simulink model "Test_apparatus"  (R2017a)
settings: Solver=VariableStepAuto  StartTime=0.0  StopTime=10  FixedStep=0.00001  RelTol=1e-3
values from neighbouring files (symbols this model uses):
  b = 0    [Oct12workspace.mat]    (also in Test_apparatus_simulation.m; custom_sim.m = 2.134608e-06)
  J = 2.134608e-05    [Oct12workspace.mat]    (also in Test_apparatus_simulation.m; custom_sim.m)
  Kd = 1000    [Oct12workspace.mat]    (also in Test_apparatus_simulation.m = dd; bilat_teleop_time_delay_params.m = 0; custom_sim.m = 35; ode45_sim.m = 0)
  Ke = 0.142826110455    [Oct12workspace.mat]    (also in Test_apparatus_simulation.m; bilat_teleop_multiDOF_params.m = [0 0; 0 0]; sampled_data_bilat_teleop_tavakoli_params.m = 0; sampled_data_bilat_teleop_time_delay_params.m = 0)
  Kp = 10000    [Oct12workspace.mat]    (also in Test_apparatus_simulation.m = pp; bilat_teleop_time_delay_params.m = 0; custom_sim.m = 100; ode45_sim.m = 100)
  KpC = 375    [Oct12workspace.mat]    (also in Test_apparatus_simulation.m; custom_sim.m = 1)
  Kt = 0.0194    [Oct12workspace.mat]    (also in Test_apparatus_simulation.m)
  L = 8.5e-05    [Oct12workspace.mat]    (also in Test_apparatus_simulation.m; custom_sim.m)
  R = 0.314    [Oct12workspace.mat]    (also in Test_apparatus_simulation.m; custom_sim.m)
  Tcontrol = 0.001    [Oct12workspace.mat]    (also in Test_apparatus_simulation.m)
  VScale = 57.2957795131    [Oct12workspace.mat]    (also in Test_apparatus_simulation.m)
  XScale = 57.2957795131    [Oct12workspace.mat]    (also in Test_apparatus_simulation.m)
libraries: simulink x3
settings Model: Creator=sansh  LastModifiedBy=salou

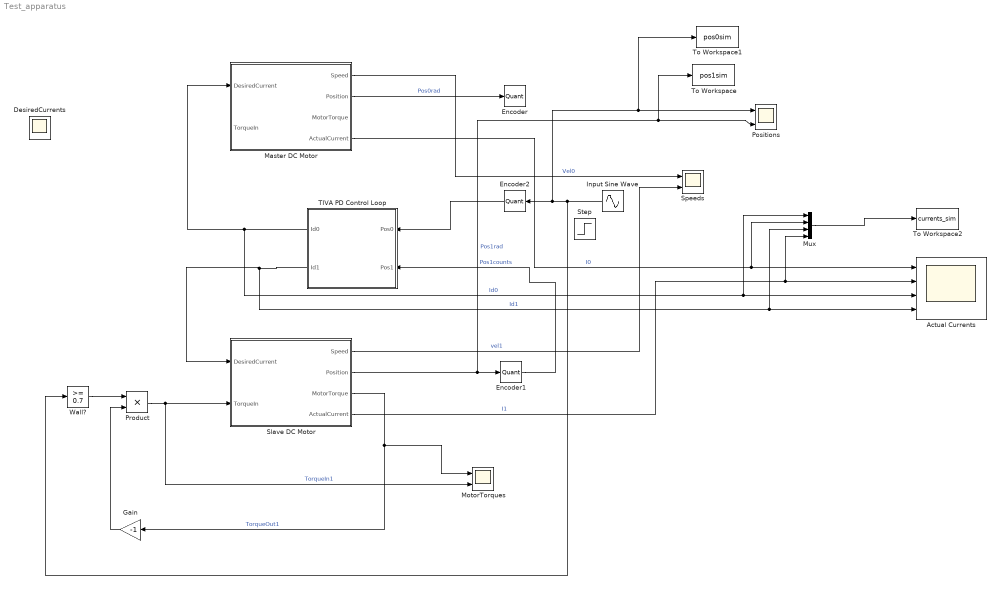
== system Test_apparatus ==
  Actual Currents : Scope  NumInputPorts=4
  DesiredCurrents : Scope
  Encoder : Quantizer  QuantizationInterval=(2*pi)/8192
  Encoder1 : Quantizer  QuantizationInterval=(2*pi)/8192
  Encoder2 : Quantizer  QuantizationInterval=(2*pi)/8192
  Gain : Gain  Gain=-1
  Input Sine Wave : Sin  SampleTime=0
  Master DC Motor : Subsystem
  MotorTorques : Scope  NumInputPorts=2
  Mux : Mux
  Positions : Scope  NumInputPorts=2
  Product : Product
  Slave DC Motor : Subsystem
  Speeds : Scope  NumInputPorts=2
  Step : Step  SampleTime=0
  TIVA PD Control Loop : Subsystem
  To Workspace : ToWorkspace  VariableName=pos1sim  SaveFormat=Timeseries  SampleTime=-1
  To Workspace1 : ToWorkspace  VariableName=pos0sim  SaveFormat=Timeseries  SampleTime=-1
  To Workspace2 : ToWorkspace  VariableName=currents_sim  SaveFormat=Timeseries  SampleTime=-1
  Wall? : simulink/Logic and Bit Operations/Compare To Constant  relop=>=  const=0.7  OutDataTypeStr=uint8
  wires:
  Master DC Motor/2(Position) -> Encoder/1  "Pos0rad"
  Slave DC Motor/2(Position) -> To Workspace/1, Positions/2, Encoder1/1  "Pos1rad"
  Encoder1/1 -> TIVA PD Control Loop/2(Pos1)  "Pos1counts"
  TIVA PD Control Loop/1(Id0) -> Mux/1, Actual Currents/3, Master DC Motor/1(DesiredCurrent)  "Id0"
  TIVA PD Control Loop/2(Id1) -> Slave DC Motor/1(DesiredCurrent), Mux/3, Actual Currents/4  "Id1"
  Input Sine Wave/1 -> Wall?/1, To Workspace1/1, Positions/1, Encoder2/1
  Encoder2/1 -> TIVA PD Control Loop/1(Pos0)
  Slave DC Motor/1(Speed) -> Speeds/2  "vel1"
  Master DC Motor/4(ActualCurrent) -> Mux/2, Actual Currents/1  "I0"
  Slave DC Motor/4(ActualCurrent) -> Mux/4, Actual Currents/2  "I1"
  Master DC Motor/1(Speed) -> Speeds/1  "Vel0"
  Mux/1 -> To Workspace2/1
  Wall?/1 -> Product/1
  Slave DC Motor/3(MotorTorque) -> MotorTorques/1, Gain/1  "TorqueOut1"
  Product/1 -> Slave DC Motor/2(TorqueIn), MotorTorques/2  "TorqueIn1"
  Gain/1 -> Product/2

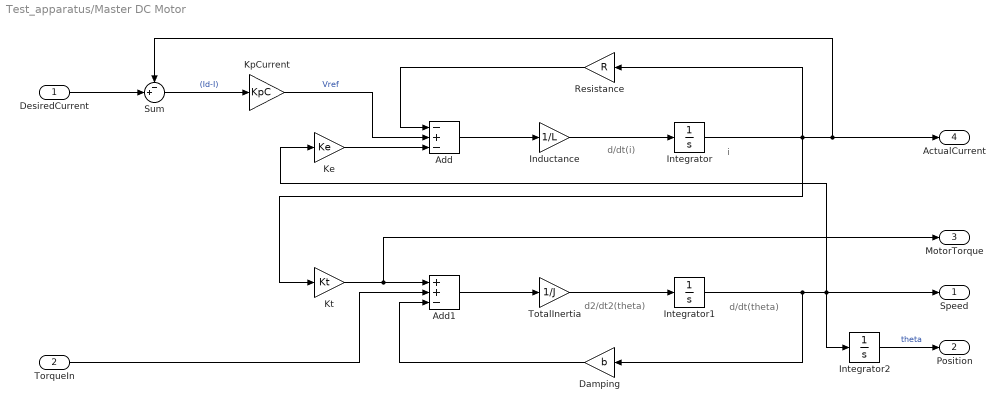
== system Test_apparatus/Master DC Motor ==
  note: i
  note: d/dt(i)
  note: d/dt(theta)
  note: d2/dt2(theta)
  DesiredCurrent : Inport
  TorqueIn : Inport  Port=2
  Add : Sum  Inputs=-+-
  Add1 : Sum  Inputs=++-
  Damping : Gain  Gain=b
  Inductance : Gain  Gain=1/L
  Integrator : Integrator
  Integrator1 : Integrator
  Integrator2 : Integrator
  Ke : Gain  Gain=Ke
  KpCurrent : Gain  Gain=KpC
  Kt : Gain  Gain=Kt
  Resistance : Gain  Gain=R
  Sum : Sum  Inputs=-+|
  TotalInertia : Gain  Gain=1/J
  Speed : Outport
  Position : Outport  Port=2
  MotorTorque : Outport  Port=3
  ActualCurrent : Outport  Port=4
  wires:
  Inductance/1 -> Integrator/1
  Integrator1/1 -> Damping/1, Integrator2/1, Speed/1, Ke/1
  TotalInertia/1 -> Integrator1/1
  Integrator/1 -> ActualCurrent/1, Sum/1, Resistance/1, Kt/1
  Kt/1 -> MotorTorque/1, Add1/1
  KpCurrent/1 -> Add/2  "Vref"
  Resistance/1 -> Add/1
  Damping/1 -> Add1/3
  Ke/1 -> Add/3
  Add/1 -> Inductance/1
  Add1/1 -> TotalInertia/1
  Integrator2/1 -> Position/1  "theta"
  DesiredCurrent/1 -> Sum/2
  Sum/1 -> KpCurrent/1  "(Id-I)"
  TorqueIn/1 -> Add1/2

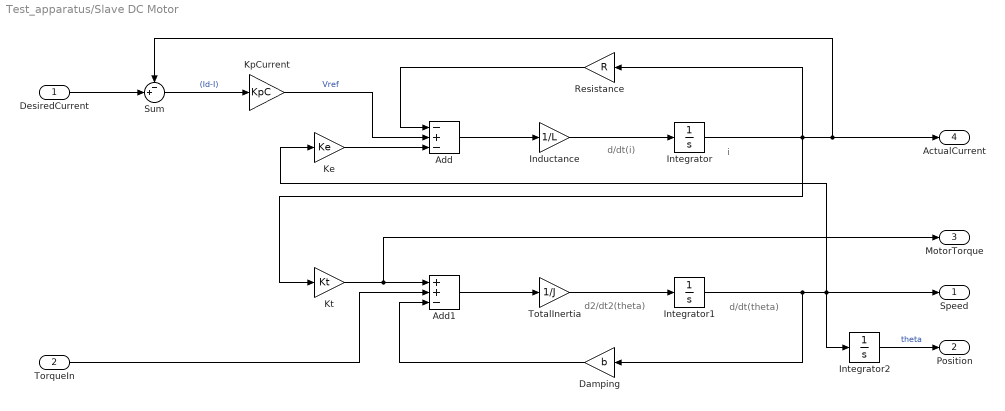
== system Test_apparatus/Slave DC Motor ==
  note: i
  note: d/dt(i)
  note: d/dt(theta)
  note: d2/dt2(theta)
  DesiredCurrent : Inport
  TorqueIn : Inport  Port=2
  Add : Sum  Inputs=-+-
  Add1 : Sum  Inputs=++-
  Damping : Gain  Gain=b
  Inductance : Gain  Gain=1/L
  Integrator : Integrator
  Integrator1 : Integrator
  Integrator2 : Integrator
  Ke : Gain  Gain=Ke
  KpCurrent : Gain  Gain=KpC
  Kt : Gain  Gain=Kt
  Resistance : Gain  Gain=R
  Sum : Sum  Inputs=-+|
  TotalInertia : Gain  Gain=1/J
  Speed : Outport
  Position : Outport  Port=2
  MotorTorque : Outport  Port=3
  ActualCurrent : Outport  Port=4
  wires:
  Inductance/1 -> Integrator/1
  Integrator1/1 -> Damping/1, Integrator2/1, Speed/1, Ke/1
  TotalInertia/1 -> Integrator1/1
  Integrator/1 -> ActualCurrent/1, Sum/1, Resistance/1, Kt/1
  Kt/1 -> MotorTorque/1, Add1/1
  KpCurrent/1 -> Add/2  "Vref"
  Resistance/1 -> Add/1
  Damping/1 -> Add1/3
  Ke/1 -> Add/3
  Add/1 -> Inductance/1
  Add1/1 -> TotalInertia/1
  Integrator2/1 -> Position/1  "theta"
  DesiredCurrent/1 -> Sum/2
  Sum/1 -> KpCurrent/1  "(Id-I)"
  TorqueIn/1 -> Add1/2

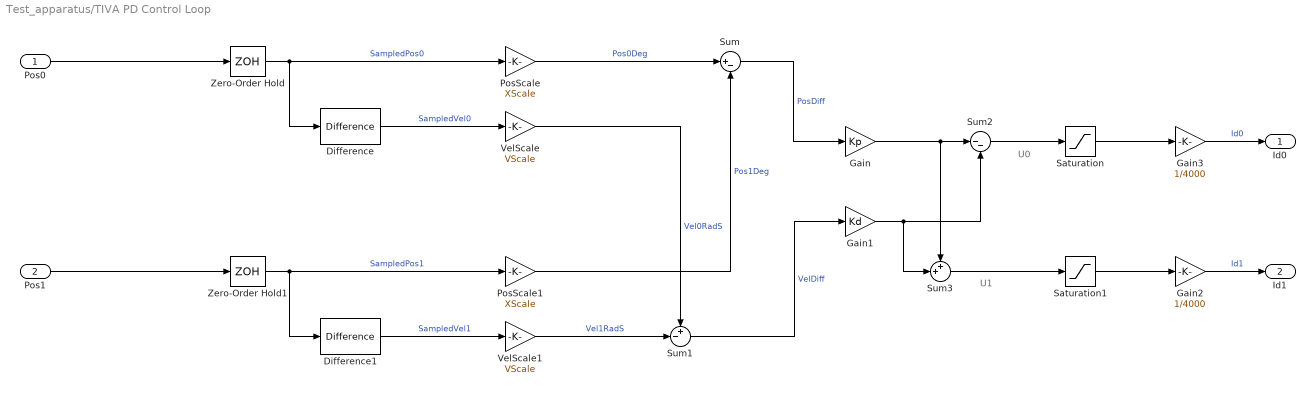
== system Test_apparatus/TIVA PD Control Loop ==
  note: U1
  note: U0
  Pos0 : Inport
  Pos1 : Inport  Port=2
  Difference : simulink/Discrete/Difference  ICPrevInput=0.0  OutMin=[]  OutMax=[]  OutDataType=fixdt(1, 16)  OutScaling=2^-10  DoSatur=off
  Difference1 : simulink/Discrete/Difference  ICPrevInput=0.0  OutMin=[]  OutMax=[]  OutDataType=fixdt(1, 16)  OutScaling=2^-10  DoSatur=off
  Gain : Gain  Gain=Kp
  Gain1 : Gain  Gain=Kd
  Gain2 : Gain  Gain=1/4000
  Gain3 : Gain  Gain=1/4000
  PosScale : Gain  Gain=XScale
  PosScale1 : Gain  Gain=XScale
  Saturation : Saturate  UpperLimit=4000  LowerLimit=-4000
  Saturation1 : Saturate  UpperLimit=4000  LowerLimit=-4000
  Sum : Sum  Inputs=|+-
  Sum1 : Sum  Inputs=+-|
  Sum2 : Sum  Inputs=|--
  Sum3 : Sum  Inputs=++|
  VelScale : Gain  Gain=VScale
  VelScale1 : Gain  Gain=VScale
  Zero-Order Hold : ZeroOrderHold  SampleTime=Tcontrol
  Zero-Order Hold1 : ZeroOrderHold  SampleTime=Tcontrol
  Id0 : Outport
  Id1 : Outport  Port=2
  wires:
  Sum/1 -> Gain/1  "PosDiff"
  Saturation/1 -> Gain3/1
  PosScale/1 -> Sum/1  "Pos0Deg"
  Pos0/1 -> Zero-Order Hold/1
  Saturation1/1 -> Gain2/1
  Zero-Order Hold/1 -> Difference/1, PosScale/1  "SampledPos0"
  Difference/1 -> VelScale/1  "SampledVel0"
  Sum1/1 -> Gain1/1  "VelDiff"
  VelScale/1 -> Sum1/1  "Vel0RadS"
  Sum2/1 -> Saturation/1
  Gain3/1 -> Id0/1  "Id0"
  Gain1/1 -> Sum2/2, Sum3/2
  Gain2/1 -> Id1/1  "Id1"
  PosScale1/1 -> Sum/2  "Pos1Deg"
  Pos1/1 -> Zero-Order Hold1/1
  Zero-Order Hold1/1 -> Difference1/1, PosScale1/1  "SampledPos1"
  Difference1/1 -> VelScale1/1  "SampledVel1"
  VelScale1/1 -> Sum1/2  "Vel1RadS"
  Gain/1 -> Sum3/1, Sum2/1
  Sum3/1 -> Saturation1/1
